simulink model "BasicPWM"  (R2018a)
settings: Solver=VariableStepAuto  StartTime=0.0  StopTime=1  RelTol=1e-3
libraries: simulink x2
settings Model: Creator=enes_  LastModifiedBy=enes_

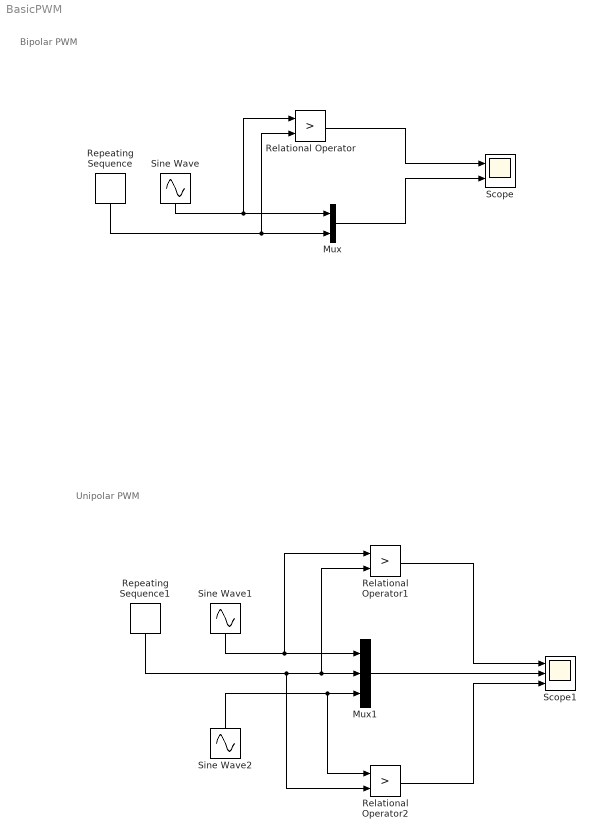
== system BasicPWM ==
  note: Unipolar PWM
  note: Bipolar PWM
  Mux : Mux  Inputs=2
  Mux1 : Mux  Inputs=3
  Relational Operator : RelationalOperator  Operator=>  OutDataTypeStr=boolean  RndMeth=Simplest
  Relational Operator1 : RelationalOperator  Operator=>  OutDataTypeStr=boolean  RndMeth=Simplest
  Relational Operator2 : RelationalOperator  Operator=>  OutDataTypeStr=boolean  RndMeth=Simplest
  Repeating Sequence : simulink/Sources/Repeating Sequence  rep_seq_t=[0 1 2 3 4]*(1/40000)  rep_seq_y=[-1 1 -1 1 -1]*(5)
  Repeating Sequence1 : simulink/Sources/Repeating Sequence  rep_seq_t=[0 1 2 3 4]*1/40000  rep_seq_y=[-1 1 -1 1 -1]*5
  Scope : Scope  NumInputPorts=2
  Scope1 : Scope  NumInputPorts=3
  Sine Wave : Sin  Amplitude=4  Frequency=2*pi*50  SampleTime=1/80000
  Sine Wave1 : Sin  Amplitude=4  Frequency=2*pi*50  SampleTime=0
  Sine Wave2 : Sin  Amplitude=4  Frequency=2*pi*50  Phase=pi  SampleTime=0
  wires:
  Sine Wave/1 -> Relational Operator/1, Mux/1
  Repeating Sequence/1 -> Relational Operator/2, Mux/2
  Relational Operator/1 -> Scope/1
  Mux/1 -> Scope/2
  Sine Wave1/1 -> Mux1/1, Relational Operator1/1
  Sine Wave2/1 -> Relational Operator2/1, Mux1/3
  Repeating Sequence1/1 -> Mux1/2, Relational Operator1/2, Relational Operator2/2
  Relational Operator1/1 -> Scope1/1
  Mux1/1 -> Scope1/2
  Relational Operator2/1 -> Scope1/3
